simulink model "warplab_mimo_4x4_unconverted_backup"  (Simulink 6.5)
settings: Solver=ode45  StartTime=0.0  StopTime=20000  RelTol=1e-3
libraries: xbsIndex_r4 x197, WARP_Blockset x16
(part 1 of 2)
settings Model: Creator=Melissa.Duarte  LastModifiedBy=melissa.duarte
settings DebuggingCC: MultiTaskDSMMsg=warning  MultiTaskCondExecSysMsg=none
settings RTWCC: IncludeERTFirstTime=on

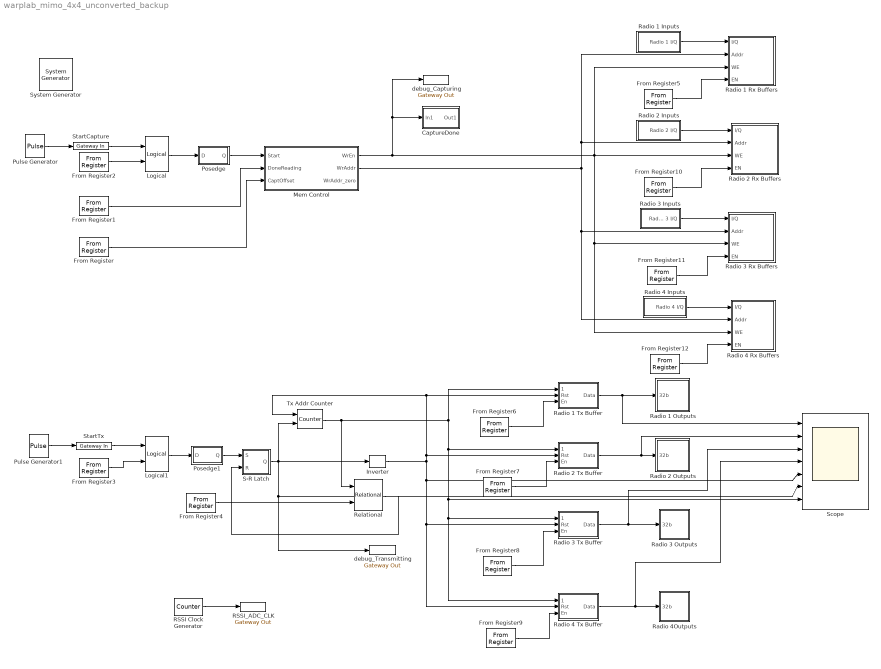
== system warplab_mimo_4x4_unconverted_backup ==
  " System Generator" : xbsIndex_r4/ System Generator  Tag=genX  SystemSampleTime=-1  xilinxfamily=Virtex4  part=xc4vsx35  speed=-10  package=ff668  synthesis_tool=XST  directory=./netlist  testbench=off  simulink_period=1  sysclk_period=10  incr_netlist=off  trim_vbits=Everywhere in SubSystem  dbl_ovrd=According to Block Masks  core_generation=According to Block Masks  run_coregen=off  deprecated_control=off  eval_field=0  block_type=sysgen
      settings: block_version=8.2
  CaptureDone : Subsystem
  From Register : xbsIndex_r4/From Register  shared_memory_name='CaptOffset'  init=100  period=1  ownership=Locally owned and initialized  arith_type=Unsigned  n_bits=14  bin_pt=0  dbl_ovrd=off  block_type=fromreg
      settings: AttributesFormatString=CaptOffset\n<< %<shared_memory_name> >>  infoedit="Register block that reads data to a shared memory register.  Delay of one sample period."  block_version=8.2
  From Register1 : xbsIndex_r4/From Register  shared_memory_name='DoneReading'  init=0  period=1  ownership=Locally owned and initialized  arith_type=Unsigned  n_bits=1  bin_pt=0  dbl_ovrd=off  block_type=fromreg
      settings: AttributesFormatString=DoneReading\n<< %<shared_memory_name> >>  infoedit="Register block that reads data to a shared memory register.  Delay of one sample period."  block_version=8.2
  From Register10 : xbsIndex_r4/From Register  shared_memory_name='RADIO2RXBUFF_RXEN'  init=0  period=1  ownership=Locally owned and initialized  arith_type=Unsigned  n_bits=1  bin_pt=0  dbl_ovrd=off  block_type=fromreg
      settings: AttributesFormatString=RADIO2RXBUFF_RXEN\n<< %<shared_memory_name> >>  infoedit="Register block that reads data to a shared memory register.  Delay of one sample period."  block_version=8.2
  From Register11 : xbsIndex_r4/From Register  shared_memory_name='RADIO3RXBUFF_RXEN'  init=0  period=1  ownership=Locally owned and initialized  arith_type=Unsigned  n_bits=1  bin_pt=0  dbl_ovrd=off  block_type=fromreg
      settings: AttributesFormatString=RADIO3RXBUFF_RXEN\n<< %<shared_memory_name> >>  infoedit="Register block that reads data to a shared memory register.  Delay of one sample period."  block_version=8.2
  From Register12 : xbsIndex_r4/From Register  shared_memory_name='RADIO4RXBUFF_RXEN'  init=0  period=1  ownership=Locally owned and initialized  arith_type=Unsigned  n_bits=1  bin_pt=0  dbl_ovrd=off  block_type=fromreg
      settings: AttributesFormatString=RADIO4RXBUFF_RXEN\n<< %<shared_memory_name> >>  infoedit="Register block that reads data to a shared memory register.  Delay of one sample period."  block_version=8.2
  From Register2 : xbsIndex_r4/From Register  shared_memory_name='StartCapture'  init=0  period=1  ownership=Locally owned and initialized  arith_type=Unsigned  n_bits=1  bin_pt=0  dbl_ovrd=off  block_type=fromreg
      settings: AttributesFormatString=StartCapture\n<< %<shared_memory_name> >>  infoedit="Register block that reads data to a shared memory register.  Delay of one sample period."  block_version=8.2
  From Register3 : xbsIndex_r4/From Register  shared_memory_name='StartTx'  init=0  period=1  ownership=Locally owned and initialized  arith_type=Unsigned  n_bits=1  bin_pt=0  dbl_ovrd=off  block_type=fromreg
      settings: AttributesFormatString=StartTx\n<< %<shared_memory_name> >>  infoedit="Register block that reads data to a shared memory register.  Delay of one sample period."  block_version=8.2
  From Register4 : xbsIndex_r4/From Register  shared_memory_name='TxLength'  init=2^14-1  period=1  ownership=Locally owned and initialized  arith_type=Unsigned  n_bits=14  bin_pt=0  dbl_ovrd=off  block_type=fromreg
      settings: AttributesFormatString=TxLength\n<< %<shared_memory_name> >>  infoedit="Register block that reads data to a shared memory register.  Delay of one sample period."  block_version=8.2
  From Register5 : xbsIndex_r4/From Register  shared_memory_name='RADIO1RXBUFF_RXEN'  init=0  period=1  ownership=Locally owned and initialized  arith_type=Unsigned  n_bits=1  bin_pt=0  dbl_ovrd=off  block_type=fromreg
      settings: AttributesFormatString=RADIO1RXBUFF_RXEN\n<< %<shared_memory_name> >>  infoedit="Register block that reads data to a shared memory register.  Delay of one sample period."  block_version=8.2
  From Register6 : xbsIndex_r4/From Register  shared_memory_name='RADIO1TXBUFF_TXEN'  init=0  period=1  ownership=Locally owned and initialized  arith_type=Unsigned  n_bits=1  bin_pt=0  dbl_ovrd=off  block_type=fromreg
      settings: AttributesFormatString=RADIO1TXBUFF_TXEN\n<< %<shared_memory_name> >>  infoedit="Register block that reads data to a shared memory register.  Delay of one sample period."  block_version=8.2
  From Register7 : xbsIndex_r4/From Register  shared_memory_name='RADIO2TXBUFF_TXEN'  init=0  period=1  ownership=Locally owned and initialized  arith_type=Unsigned  n_bits=1  bin_pt=0  dbl_ovrd=off  block_type=fromreg
      settings: AttributesFormatString=RADIO2TXBUFF_TXEN\n<< %<shared_memory_name> >>  infoedit="Register block that reads data to a shared memory register.  Delay of one sample period."  block_version=8.2
  From Register8 : xbsIndex_r4/From Register  shared_memory_name='RADIO3TXBUFF_TXEN'  init=0  period=1  ownership=Locally owned and initialized  arith_type=Unsigned  n_bits=1  bin_pt=0  dbl_ovrd=off  block_type=fromreg
      settings: AttributesFormatString=RADIO3TXBUFF_TXEN\n<< %<shared_memory_name> >>  infoedit="Register block that reads data to a shared memory register.  Delay of one sample period."  block_version=8.2
  From Register9 : xbsIndex_r4/From Register  shared_memory_name='RADIO4TXBUFF_TXEN'  init=0  period=1  ownership=Locally owned and initialized  arith_type=Unsigned  n_bits=1  bin_pt=0  dbl_ovrd=off  block_type=fromreg
      settings: AttributesFormatString=RADIO4TXBUFF_TXEN\n<< %<shared_memory_name> >>  infoedit="Register block that reads data to a shared memory register.  Delay of one sample period."  block_version=8.2
  Inverter : xbsIndex_r4/Inverter  en=off  latency=0  dbl_ovrd=off  block_type=inv
      settings: block_version=8.2
  Logical : xbsIndex_r4/Logical  logical_function=OR  inputs=2  en=off  latency=0  precision=Full  arith_type=Unsigned  n_bits=16  bin_pt=0  align_bp=on  dbl_ovrd=off  block_type=logical
      settings: block_version=8.2
  Logical1 : xbsIndex_r4/Logical  logical_function=OR  inputs=2  en=off  latency=0  precision=Full  arith_type=Unsigned  n_bits=16  bin_pt=0  align_bp=on  dbl_ovrd=off  block_type=logical
      settings: block_version=8.2
  Mem Control : Subsystem
  Posedge : Subsystem
  Posedge1 : Subsystem
  Pulse Generator : DiscretePulseGenerator  Period=1000000  PulseWidth=50  PhaseDelay=2
  Pulse Generator1 : DiscretePulseGenerator  Period=1000000  PulseWidth=50  PhaseDelay=2
  RSSI Clock Generator : xbsIndex_r4/Counter  cnt_type=Free Running  cnt_to=Inf  operation=Up  start_count=0  cnt_by_val=1  arith_type=Unsigned  n_bits=1  bin_pt=0  load_pin=off  rst=off  en=off  explicit_period=on  period=2  dbl_ovrd=off  use_behavioral_HDL=off  use_rpm=off  block_type=counter
      settings: block_version=VER_STRING_GOES_HERE
  RSSI_ADC_CLK : xbsIndex_r4/Gateway Out  hdl_port=on  timing_constraint=None  locs_specified=off  LOCs={}  block_type=gatewayout
      settings: infoedit="Gateway out block.  Converts Xilinx fixed point inputs into ouputs of type Simulink integer, double, or fixed point.<P><P>Hardware notes:  In hardware these blocks become top level output ports or are discarded, depending on how they are configured."  block_version=8.2
  Radio 1 Rx Buffers : Subsystem
  Radio 1 Tx Buffer : Subsystem
  Radio 1 Inputs : Subsystem
  Radio 1 Outputs : Subsystem
  Radio 2 Rx Buffers : Subsystem
  Radio 2 Tx Buffer : Subsystem
  Radio 2 Inputs : Subsystem
  Radio 2 Outputs : Subsystem
  Radio 3 Rx Buffers : Subsystem
  Radio 3 Tx Buffer : Subsystem
  Radio 3 Inputs : Subsystem
  Radio 3 Outputs : Subsystem
  Radio 4 Rx Buffers : Subsystem
  Radio 4 Tx Buffer : Subsystem
  Radio 4 Inputs : Subsystem
  Radio 4Outputs : Subsystem
  Relational : xbsIndex_r4/Relational  mode=a>=b  en=off  latency=0  dbl_ovrd=off  block_type=relational
      settings: block_version=8.2
  S-R Latch : Subsystem
  Scope : Scope  NumInputPorts=7
      settings: YMin=-5~-5~-5~-5~-5~-5~-5  YMax=5~5~5~5~5~5~5  SaveName=ScopeData2  MaxDataPoints=50000
  StartCapture : xbsIndex_r4/Gateway In  arith_type=Unsigned  n_bits=1  bin_pt=0  quantization="Round  (unbiased: +/- Inf)"  overflow=Saturate  period=1  dbl_ovrd=off  timing_constraint=None  locs_specified=off  LOCs={}  block_type=gatewayin
      settings: infoedit="Gateway in block.  Converts inputs of type Simulink integer, double and fixed point to  Xilinx fixed point type.<P><P>Hardware notes:  In hardware these blocks become top level input ports."  block_version=VER_STRING_GOES_HERE
  StartTx : xbsIndex_r4/Gateway In  arith_type=Unsigned  n_bits=1  bin_pt=0  quantization="Round  (unbiased: +/- Inf)"  overflow=Saturate  period=1  dbl_ovrd=off  timing_constraint=None  locs_specified=off  LOCs={}  block_type=gatewayin
      settings: infoedit="Gateway in block.  Converts inputs of type Simulink integer, double and fixed point to  Xilinx fixed point type.<P><P>Hardware notes:  In hardware these blocks become top level input ports."  block_version=VER_STRING_GOES_HERE
  Tx Addr Counter : xbsIndex_r4/Counter  cnt_type=Free Running  cnt_to=Inf  operation=Up  start_count=0  cnt_by_val=1  arith_type=Unsigned  n_bits=14  bin_pt=0  load_pin=off  rst=on  en=on  explicit_period=off  period=1  dbl_ovrd=off  use_behavioral_HDL=off  use_rpm=off  block_type=counter
      settings: block_version=8.2
  debug_Capturing : xbsIndex_r4/Gateway Out  hdl_port=on  timing_constraint=None  locs_specified=off  LOCs={}  block_type=gatewayout
      settings: infoedit="Gateway out block.  Converts Xilinx fixed point inputs into ouputs of type Simulink integer, double, or fixed point.<P><P>Hardware notes:  In hardware these blocks become top level output ports or are discarded, depending on how they are configured."  block_version=8.2
  debug_Transmitting : xbsIndex_r4/Gateway Out  hdl_port=on  timing_constraint=None  locs_specified=off  LOCs={}  block_type=gatewayout
      settings: infoedit="Gateway out block.  Converts Xilinx fixed point inputs into ouputs of type Simulink integer, double, or fixed point.<P><P>Hardware notes:  In hardware these blocks become top level output ports or are discarded, depending on how they are configured."  block_version=8.2
  wires:
  Posedge/1(Q) -> Mem Control/1(Start)
  From Register/1 -> Mem Control/3(CaptOffset)
  From Register1/1 -> Mem Control/2(DoneReading)
  Pulse Generator/1 -> StartCapture/1
  From Register2/1 -> Logical/2
  Logical/1 -> Posedge/1(D)
  StartCapture/1 -> Logical/1
  Tx Addr Counter/1 -> Relational/1, Radio 1 Tx Buffer/1(RdAddr), Radio 2 Tx Buffer/1(RdAddr), Radio 3 Tx Buffer/1(RdAddr), Radio 4 Tx Buffer/1(RdAddr), Scope/7
  S-R Latch/1(Q) -> Inverter/1, Tx Addr Counter/2, debug_Transmitting/1, Scope/6
  From Register4/1 -> Relational/2
  Relational/1 -> S-R Latch/2(R)
  Inverter/1 -> Radio 1 Tx Buffer/2(Rst), Tx Addr Counter/1, Radio 2 Tx Buffer/2(Rst), Radio 3 Tx Buffer/2(Rst), Radio 4 Tx Buffer/2(Rst), Scope/5
  Radio 1 Inputs/1(Radio 1 I/Q) -> Radio 1 Rx Buffers/1(I/Q)
  RSSI Clock Generator/1 -> RSSI_ADC_CLK/1
  Posedge1/1(Q) -> S-R Latch/1(S)
  Radio 2 Inputs/1(Radio 2 I/Q) -> Radio 2 Rx Buffers/1(I/Q)
  Radio 4 Inputs/1(Radio 4 I/Q) -> Radio 4 Rx Buffers/1(I/Q)
  Radio 3 Inputs/1(Radio 3 I/Q) -> Radio 3 Rx Buffers/1(I/Q)
  Pulse Generator1/1 -> StartTx/1
  StartTx/1 -> Logical1/1
  Logical1/1 -> Posedge1/1(D)
  From Register3/1 -> Logical1/2
  Mem Control/1(WrEn) -> CaptureDone/1(In1), debug_Capturing/1, Radio 2 Rx Buffers/3(WE), Radio 1 Rx Buffers/3(WE), Radio 3 Rx Buffers/3(WE), Radio 4 Rx Buffers/3(WE)
  Mem Control/2(WrAddr) -> Radio 1 Rx Buffers/2(Addr), Radio 2 Rx Buffers/2(Addr), Radio 3 Rx Buffers/2(Addr), Radio 4 Rx Buffers/2(Addr)
  From Register6/1 -> Radio 1 Tx Buffer/3(En)
  From Register7/1 -> Radio 2 Tx Buffer/3(En)
  From Register8/1 -> Radio 3 Tx Buffer/3(En)
  From Register9/1 -> Radio 4 Tx Buffer/3(En)
  From Register5/1 -> Radio 1 Rx Buffers/4(EN)
  From Register10/1 -> Radio 2 Rx Buffers/4(EN)
  From Register11/1 -> Radio 3 Rx Buffers/4(EN)
  From Register12/1 -> Radio 4 Rx Buffers/4(EN)
  Radio 1 Tx Buffer/1(Data) -> Radio 1 Outputs/1(32b), Scope/1
  Radio 2 Tx Buffer/1(Data) -> Radio 2 Outputs/1(32b), Scope/2
  Radio 3 Tx Buffer/1(Data) -> Radio 3 Outputs/1(32b), Scope/3
  Radio 4 Tx Buffer/1(Data) -> Radio 4Outputs/1(32b), Scope/4

== system warplab_mimo_4x4_unconverted_backup/CaptureDone ==
  In1 : Inport
  Inverter1 : xbsIndex_r4/Inverter  en=off  latency=0  dbl_ovrd=off  block_type=inv
      settings: block_version=8.2
  To Register : xbsIndex_r4/To Register  shared_memory_name='CaptureDone'  init=0  ownership=Locally owned and initialized  explicit_data_type=off  arith_type="Signed  (2's comp)"  n_bits=16  bin_pt=14  dbl_ovrd=off  block_type=toreg
      settings: AttributesFormatString=CaptureDone\n<< %<shared_memory_name> >>  infoedit="Register block that writes data to a shared memory register.  Delay of one sample period."  block_version=8.2
  zero3 : xbsIndex_r4/Constant  arith_type=Boolean  const=1  n_bits=1  bin_pt=0  explicit_period=off  period=1  equ=P=C  opselect=C  inp2=PCIN>>17  opr=+  inp1=P  carry=CIN  dbl_ovrd=off  block_type=constant
      settings: block_version=VER_STRING_GOES_HERE
  Out1 : Outport
  wires:
  zero3/1 -> To Register/2
  Inverter1/1 -> To Register/1
  In1/1 -> Inverter1/1
  To Register/1 -> Out1/1

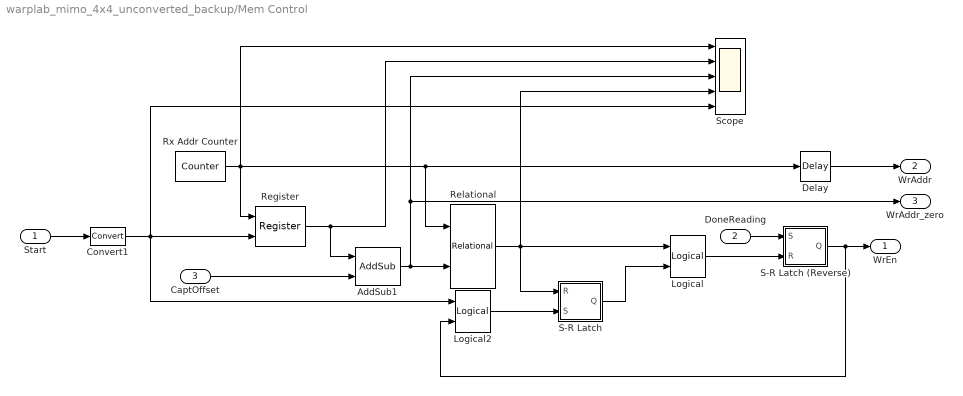
== system warplab_mimo_4x4_unconverted_backup/Mem Control ==
  Start : Inport
  DoneReading : Inport  Port=2
  CaptOffset : Inport  Port=3
  AddSub1 : xbsIndex_r4/AddSub  mode=Subtraction  use_carryin=off  use_carryout=off  en=off  latency=0  precision=User Defined  arith_type=Unsigned  n_bits=14  bin_pt=0  quantization=Truncate  overflow=Wrap  dbl_ovrd=off  use_behavioral_HDL=off  pipelined=off  use_rpm=on  block_type=addsub
      settings: block_version=8.2
  Convert1 : xbsIndex_r4/Convert  arith_type=Boolean  n_bits=16  bin_pt=14  quantization=Truncate  overflow=Wrap  latency=0  dbl_ovrd=off  pipeline=off  block_type=convert
      settings: block_version=8.2
  Delay : xbsIndex_r4/Delay  en=off  latency=1  dbl_ovrd=off  reg_retiming=off  block_type=delay
      settings: infoedit=Hardware notes: A delay line is a chain, each link of which is an SRL16 followed by a flip-flop. If register retiming is enabled, the delay line is a chain of flip-flops.  block_version=8.2
  Logical : xbsIndex_r4/Logical  logical_function=AND  inputs=2  en=off  latency=0  precision=Full  arith_type=Unsigned  n_bits=16  bin_pt=0  align_bp=on  dbl_ovrd=off  block_type=logical
      settings: block_version=8.2
  Logical2 : xbsIndex_r4/Logical  logical_function=AND  inputs=2  en=off  latency=0  precision=Full  arith_type=Unsigned  n_bits=16  bin_pt=0  align_bp=on  dbl_ovrd=off  block_type=logical
      settings: block_version=8.2
  Register : xbsIndex_r4/Register  init=0  rst=off  en=on  dbl_ovrd=off  block_type=register
      settings: block_version=8.2
  Relational : xbsIndex_r4/Relational  mode=a=b  en=off  latency=0  dbl_ovrd=off  block_type=relational
      settings: block_version=8.2
  Rx Addr Counter : xbsIndex_r4/Counter  cnt_type=Free Running  cnt_to=Inf  operation=Up  start_count=0  cnt_by_val=1  arith_type=Unsigned  n_bits=14  bin_pt=0  load_pin=off  rst=off  en=off  explicit_period=on  period=1  dbl_ovrd=off  use_behavioral_HDL=off  use_rpm=off  block_type=counter
      settings: block_version=8.2
  S-R Latch : Subsystem
  S-R Latch (Reverse) : Subsystem
  Scope : Scope  NumInputPorts=5
      settings: TimeRange=100000  YMin=0~-1~15469.8~0~-1  YMax=17500~1~17098.2~1~1
  WrEn : Outport
  WrAddr : Outport  Port=2
  WrAddr_zero : Outport  Port=3
  wires:
  CaptOffset/1 -> AddSub1/2
  Register/1 -> AddSub1/1, Scope/2
  AddSub1/1 -> Relational/2, Scope/3, WrAddr_zero/1
  DoneReading/1 -> S-R Latch (Reverse)/1(S)
  Relational/1 -> S-R Latch/1(R), Logical/1, Scope/4
  Rx Addr Counter/1 -> Scope/1, Register/1, Delay/1, Relational/1
  Start/1 -> Convert1/1
  S-R Latch (Reverse)/1(Q) -> WrEn/1, Logical2/2
  Delay/1 -> WrAddr/1
  Convert1/1 -> Register/2, Scope/5, Logical2/1
  Logical/1 -> S-R Latch (Reverse)/2(R)
  S-R Latch/1(Q) -> Logical/2
  Logical2/1 -> S-R Latch/2(S)

== system warplab_mimo_4x4_unconverted_backup/Posedge ==
  D : Inport
  Delay : xbsIndex_r4/Delay  en=off  latency=1  dbl_ovrd=off  reg_retiming=off  block_type=delay
      settings: infoedit=Hardware notes: A delay line is a chain, each link of which is an SRL16 followed by a flip-flop. If register retiming is enabled, the delay line is a chain of flip-flops.  block_version=8.2
  Inverter : xbsIndex_r4/Inverter  en=off  latency=0  dbl_ovrd=off  block_type=inv
      settings: block_version=8.2
  Logical : xbsIndex_r4/Logical  logical_function=AND  inputs=2  en=off  latency=0  precision=Full  arith_type=Unsigned  n_bits=16  bin_pt=0  align_bp=on  dbl_ovrd=off  block_type=logical
      settings: block_version=8.2
  Q : Outport
  wires:
  D/1 -> Inverter/1, Logical/1
  Inverter/1 -> Delay/1
  Delay/1 -> Logical/2
  Logical/1 -> Q/1

== system warplab_mimo_4x4_unconverted_backup/Posedge1 ==
  D : Inport
  Delay : xbsIndex_r4/Delay  en=off  latency=1  dbl_ovrd=off  reg_retiming=off  block_type=delay
      settings: infoedit=Hardware notes: A delay line is a chain, each link of which is an SRL16 followed by a flip-flop. If register retiming is enabled, the delay line is a chain of flip-flops.  block_version=8.2
  Inverter : xbsIndex_r4/Inverter  en=off  latency=0  dbl_ovrd=off  block_type=inv
      settings: block_version=8.2
  Logical : xbsIndex_r4/Logical  logical_function=AND  inputs=2  en=off  latency=0  precision=Full  arith_type=Unsigned  n_bits=16  bin_pt=0  align_bp=on  dbl_ovrd=off  block_type=logical
      settings: block_version=8.2
  Q : Outport
  wires:
  Logical/1 -> Q/1
  Delay/1 -> Logical/2
  Inverter/1 -> Delay/1
  D/1 -> Logical/1, Inverter/1

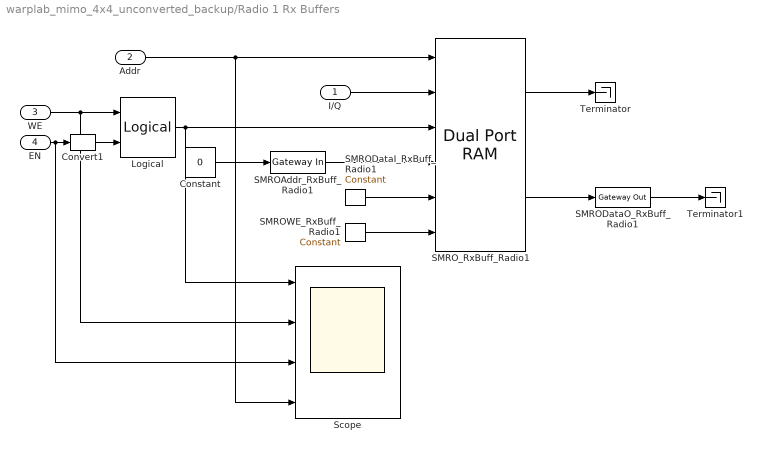
== system warplab_mimo_4x4_unconverted_backup/Radio 1 Rx Buffers ==
  I/Q : Inport
  Addr : Inport  Port=2
  WE : Inport  Port=3
  EN : Inport  Port=4
  Constant : Constant  Value=0  OutDataType=sfix(16)  ConRadixGroup=Use specified scaling  OutScaling=2^0  SampleTime=inf  FramePeriod=inf
  Convert1 : xbsIndex_r4/Convert  arith_type=Boolean  n_bits=16  bin_pt=14  quantization=Truncate  overflow=Wrap  latency=0  dbl_ovrd=off  pipeline=off  block_type=convert
      settings: block_version=8.2
  Logical : xbsIndex_r4/Logical  logical_function=AND  inputs=2  en=off  latency=0  precision=Full  arith_type=Unsigned  n_bits=16  bin_pt=0  align_bp=on  dbl_ovrd=off  block_type=logical
      settings: block_version=9.1.01
  SMROAddr_RxBuff_Radio1 : xbsIndex_r4/Gateway In  arith_type=Unsigned  n_bits=14  bin_pt=0  quantization="Round  (unbiased: +/- Inf)"  overflow=Saturate  period=1  dbl_ovrd=off  timing_constraint=None  locs_specified=off  LOCs={}  block_type=gatewayin
      settings: infoedit="Gateway in block.  Converts inputs of type Simulink integer, double and fixed point to  Xilinx fixed point type.<P><P>Hardware notes:  In hardware these blocks become top level input ports."  block_version=VER_STRING_GOES_HERE
  SMRODataI_RxBuff_Radio1 : xbsIndex_r4/Constant  arith_type=Unsigned  const=0  n_bits=32  bin_pt=0  explicit_period=off  period=1  equ=P=C  opselect=C  inp2=PCIN>>17  opr=+  inp1=P  carry=CIN  dbl_ovrd=off  block_type=constant
      settings: block_version=VER_STRING_GOES_HERE
  SMRODataO_RxBuff_Radio1 : xbsIndex_r4/Gateway Out  hdl_port=on  timing_constraint=None  locs_specified=off  LOCs={}  block_type=gatewayout
      settings: infoedit="Gateway out block.  Converts Xilinx fixed point inputs into ouputs of type Simulink integer, double, or fixed point.<P><P>Hardware notes:  In hardware these blocks become top level output ports or are discarded, depending on how they are configured."  xl_area=[0, 0, 0, 0, 0, 0, 0]  block_version=VER_STRING_GOES_HERE
  SMROWE_RxBuff_Radio1 : xbsIndex_r4/Constant  arith_type=Boolean  const=0  n_bits=3  bin_pt=0  explicit_period=off  period=1  equ=P=C  opselect=C  inp2=PCIN>>17  opr=+  inp1=P  carry=CIN  dbl_ovrd=off  block_type=constant
      settings: block_version=VER_STRING_GOES_HERE
  SMRO_RxBuff_Radio1 : xbsIndex_r4/Dual Port RAM  depth=2^14  initVector=1:2^14  distributed_mem=Block RAM  init_a=0  init_b=0  rst_a=off  rst_b=off  en_a=off  en_b=off  latency=1  write_mode_A=Read After Write  write_mode_B=Read After Write  dbl_ovrd=off  optimize=Area  use_rpm=on  block_type=dpram
      settings: block_version=VER_STRING_GOES_HERE
  Scope : Scope  NumInputPorts=4
      settings: YMin=-5~-5~-5~-5  YMax=5~5~5~5  SaveName=ScopeData3  MaxDataPoints=50000
  Terminator : Terminator
  Terminator1 : Terminator
  wires:
  I/Q/1 -> SMRO_RxBuff_Radio1/2
  Addr/1 -> SMRO_RxBuff_Radio1/1, Scope/4
  SMRODataO_RxBuff_Radio1/1 -> Terminator1/1
  SMRO_RxBuff_Radio1/1 -> Terminator/1
  SMROAddr_RxBuff_Radio1/1 -> SMRO_RxBuff_Radio1/4
  SMRO_RxBuff_Radio1/2 -> SMRODataO_RxBuff_Radio1/1
  Constant/1 -> SMROAddr_RxBuff_Radio1/1
  SMRODataI_RxBuff_Radio1/1 -> SMRO_RxBuff_Radio1/5
  SMROWE_RxBuff_Radio1/1 -> SMRO_RxBuff_Radio1/6
  Logical/1 -> SMRO_RxBuff_Radio1/3, Scope/1
  WE/1 -> Logical/1, Scope/2
  EN/1 -> Convert1/1, Scope/3
  Convert1/1 -> Logical/2

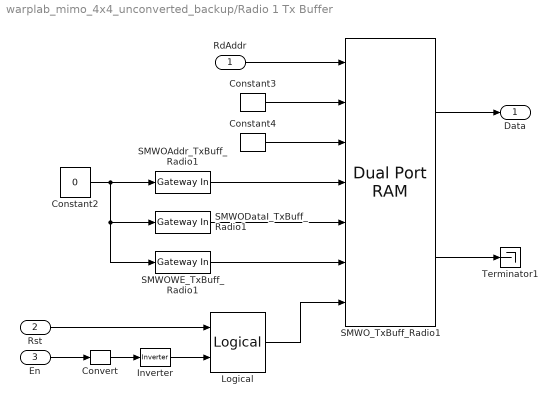
== system warplab_mimo_4x4_unconverted_backup/Radio 1 Tx Buffer ==
  RdAddr : Inport
  Rst : Inport  Port=2
  En : Inport  Port=3
  Constant2 : Constant  Value=0  OutDataType=sfix(16)  ConRadixGroup=Use specified scaling  OutScaling=2^0  SampleTime=inf  FramePeriod=inf
  Constant3 : xbsIndex_r4/Constant  arith_type=Unsigned  const=0  n_bits=32  bin_pt=0  explicit_period=off  period=1  equ=P=C  opselect=C  inp2=PCIN>>17  opr=+  inp1=P  carry=CIN  dbl_ovrd=off  block_type=constant
      settings: block_version=VER_STRING_GOES_HERE
  Constant4 : xbsIndex_r4/Constant  arith_type=Boolean  const=0  n_bits=1  bin_pt=0  explicit_period=off  period=1  equ=P=C  opselect=C  inp2=PCIN>>17  opr=+  inp1=P  carry=CIN  dbl_ovrd=off  block_type=constant
      settings: block_version=VER_STRING_GOES_HERE
  Convert : xbsIndex_r4/Convert  arith_type=Boolean  n_bits=16  bin_pt=14  quantization=Truncate  overflow=Wrap  latency=0  dbl_ovrd=off  pipeline=off  block_type=convert
      settings: block_version=8.2
  Inverter : xbsIndex_r4/Inverter  en=off  latency=0  dbl_ovrd=off  block_type=inv
      settings: block_version=9.1.01
  Logical : xbsIndex_r4/Logical  logical_function=OR  inputs=2  en=off  latency=0  precision=Full  arith_type=Unsigned  n_bits=16  bin_pt=0  align_bp=on  dbl_ovrd=off  block_type=logical
      settings: block_version=9.1.01
  SMWOAddr_TxBuff_Radio1 : xbsIndex_r4/Gateway In  arith_type=Unsigned  n_bits=14  bin_pt=0  quantization="Round  (unbiased: +/- Inf)"  overflow=Saturate  period=1  dbl_ovrd=off  timing_constraint=None  locs_specified=off  LOCs={}  block_type=gatewayin
      settings: infoedit="Gateway in block.  Converts inputs of type Simulink integer, double and fixed point to  Xilinx fixed point type.<P><P>Hardware notes:  In hardware these blocks become top level input ports."  block_version=VER_STRING_GOES_HERE
  SMWODataI_TxBuff_Radio1 : xbsIndex_r4/Gateway In  arith_type=Unsigned  n_bits=32  bin_pt=0  quantization="Round  (unbiased: +/- Inf)"  overflow=Saturate  period=1  dbl_ovrd=off  timing_constraint=None  locs_specified=off  LOCs={}  block_type=gatewayin
      settings: infoedit="Gateway in block.  Converts inputs of type Simulink integer, double and fixed point to  Xilinx fixed point type.<P><P>Hardware notes:  In hardware these blocks become top level input ports."  block_version=VER_STRING_GOES_HERE
  SMWOWE_TxBuff_Radio1 : xbsIndex_r4/Gateway In  arith_type=Boolean  n_bits=1  bin_pt=0  quantization="Round  (unbiased: +/- Inf)"  overflow=Saturate  period=1  dbl_ovrd=off  timing_constraint=None  locs_specified=off  LOCs={}  block_type=gatewayin
      settings: infoedit="Gateway in block.  Converts inputs of type Simulink integer, double and fixed point to  Xilinx fixed point type.<P><P>Hardware notes:  In hardware these blocks become top level input ports."  block_version=VER_STRING_GOES_HERE
  SMWO_TxBuff_Radio1 : xbsIndex_r4/Dual Port RAM  depth=2^14  initVector=1:2^14  distributed_mem=Block RAM  init_a=0  init_b=0  rst_a=on  rst_b=off  en_a=off  en_b=off  latency=1  write_mode_A=Read After Write  write_mode_B=Read After Write  dbl_ovrd=off  optimize=Area  use_rpm=on  block_type=dpram
      settings: block_version=VER_STRING_GOES_HERE
  Terminator1 : Terminator
  Data : Outport
  wires:
  SMWO_TxBuff_Radio1/2 -> Terminator1/1
  SMWODataI_TxBuff_Radio1/1 -> SMWO_TxBuff_Radio1/5
  SMWOWE_TxBuff_Radio1/1 -> SMWO_TxBuff_Radio1/6
  SMWOAddr_TxBuff_Radio1/1 -> SMWO_TxBuff_Radio1/4
  Constant3/1 -> SMWO_TxBuff_Radio1/2
  Constant4/1 -> SMWO_TxBuff_Radio1/3
  Constant2/1 -> SMWOAddr_TxBuff_Radio1/1, SMWODataI_TxBuff_Radio1/1, SMWOWE_TxBuff_Radio1/1
  RdAddr/1 -> SMWO_TxBuff_Radio1/1
  SMWO_TxBuff_Radio1/1 -> Data/1
  Logical/1 -> SMWO_TxBuff_Radio1/7
  Rst/1 -> Logical/1
  Inverter/1 -> Logical/2
  En/1 -> Convert/1
  Convert/1 -> Inverter/1

== system warplab_mimo_4x4_unconverted_backup/Radio 1 Inputs ==
  ADC I : Subsystem
  ADC Q : Subsystem
  Concatenates_1 : Subsystem
  Scope : Scope  NumInputPorts=3
      settings: YMin=-5~-5~-5  YMax=5~5~5
  Radio 1 I/Q : Outport
  wires:
  ADC Q/2(ADC Q) -> Concatenates_1/4(ADC_Q), Scope/2
  ADC Q/1(OTR Q) -> Concatenates_1/3(OTR_Q)
  ADC I/2(ADC I) -> Concatenates_1/2(ADC_I), Scope/1
  ADC I/1(OTR I) -> Concatenates_1/1(OTR_I)
  Concatenates_1/1(32b) -> Radio 1 I/Q/1

== system warplab_mimo_4x4_unconverted_backup/Radio 1 Outputs ==
  32b : Inport
  16LSB : xbsIndex_r4/Slice  nbits=16  boolean_output=off  mode=Lower Bit Location + Width  bit1=0  base1=MSB of Input  bit0=0  base0=LSB of Input  dbl_ovrd=off  block_type=slice
      settings: infoedit="Extracts a given range of bits from each input sample and presents it at the output.  The output type is ordinarily unsigned with binary point at zero, but can be Boolean when the slice is one bit wide.<P><P>Hardware notes: In hardware this block costs nothing."  block_version=8.2
  16MSB : xbsIndex_r4/Slice  nbits=16  boolean_output=off  mode=Upper Bit Location + Width  bit1=0  base1=MSB of Input  bit0=0  base0=LSB of Input  dbl_ovrd=off  block_type=slice
      settings: infoedit="Extracts a given range of bits from each input sample and presents it at the output.  The output type is ordinarily unsigned with binary point at zero, but can be Boolean when the slice is one bit wide.<P><P>Hardware notes: In hardware this block costs nothing."  block_version=8.2
  Radio 1 DAC I : WARP_Blockset/WARP Radio ADC//DACs/Radio 1 DAC I  SystemSampleTime=-1
  Radio 1 DAC Q : WARP_Blockset/WARP Radio ADC//DACs/Radio 1 DAC Q  SystemSampleTime=-1
  Register : xbsIndex_r4/Register  init=0  rst=off  en=off  dbl_ovrd=off  block_type=register
      settings: block_version=8.2
  Register1 : xbsIndex_r4/Register  init=0  rst=off  en=off  dbl_ovrd=off  block_type=register
      settings: block_version=8.2
  Reinterpret : xbsIndex_r4/Reinterpret  force_arith_type=on  arith_type="Signed  (2's comp)"  force_bin_pt=on  bin_pt=15  block_type=reinterpret
      settings: infoedit="Changes signal type without altering the binary representation.   You can changed the signal between signed and unsigned, and relocate the binary point.<P><P>Hardware notes: In hardware this block costs nothing.<P><P>Example:  Suppose the input is 6 bits wide, signed, with 2 fractional bits, and the output is forced to unsigned with 0 fractional bits.  Then an input of -2.0 (1110.00 in binary 2's complement) becomes an output of 56 (111000 in binary)."  block_version=8.2
  Reinterpret1 : xbsIndex_r4/Reinterpret  force_arith_type=on  arith_type="Signed  (2's comp)"  force_bin_pt=on  bin_pt=15  block_type=reinterpret
      settings: infoedit="Changes signal type without altering the binary representation.   You can changed the signal between signed and unsigned, and relocate the binary point.<P><P>Hardware notes: In hardware this block costs nothing.<P><P>Example:  Suppose the input is 6 bits wide, signed, with 2 fractional bits, and the output is forced to unsigned with 0 fractional bits.  Then an input of -2.0 (1110.00 in binary 2's complement) becomes an output of 56 (111000 in binary)."  block_version=8.2
  Terminator1 : Terminator
  Terminator2 : Terminator
  wires:
  Register1/1 -> Radio 1 DAC Q/1
  Register/1 -> Radio 1 DAC I/1
  16MSB/1 -> Reinterpret/1
  16LSB/1 -> Reinterpret1/1
  Reinterpret/1 -> Register/1
  Reinterpret1/1 -> Register1/1
  Radio 1 DAC I/1 -> Terminator1/1
  Radio 1 DAC Q/1 -> Terminator2/1
  32b/1 -> 16LSB/1, 16MSB/1

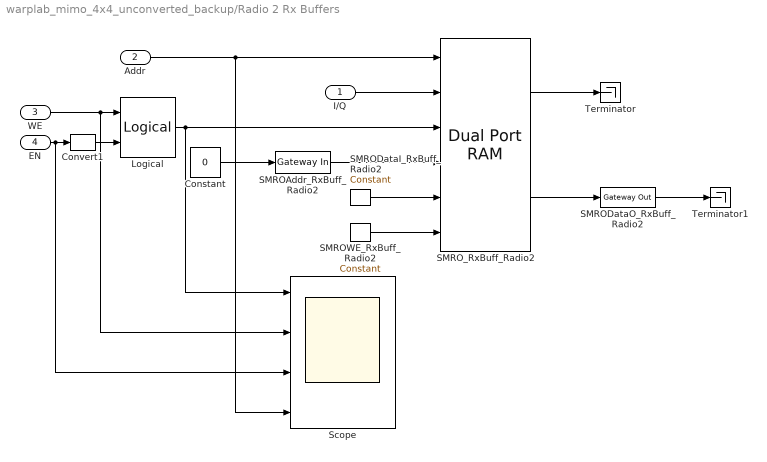
== system warplab_mimo_4x4_unconverted_backup/Radio 2 Rx Buffers ==
  I/Q : Inport
  Addr : Inport  Port=2
  WE : Inport  Port=3
  EN : Inport  Port=4
  Constant : Constant  Value=0  OutDataType=sfix(16)  ConRadixGroup=Use specified scaling  OutScaling=2^0  SampleTime=inf  FramePeriod=inf
  Convert1 : xbsIndex_r4/Convert  arith_type=Boolean  n_bits=16  bin_pt=14  quantization=Truncate  overflow=Wrap  latency=0  dbl_ovrd=off  pipeline=off  block_type=convert
      settings: block_version=8.2
  Logical : xbsIndex_r4/Logical  logical_function=AND  inputs=2  en=off  latency=0  precision=Full  arith_type=Unsigned  n_bits=16  bin_pt=0  align_bp=on  dbl_ovrd=off  block_type=logical
      settings: block_version=9.1.01
  SMROAddr_RxBuff_Radio2 : xbsIndex_r4/Gateway In  arith_type=Unsigned  n_bits=14  bin_pt=0  quantization="Round  (unbiased: +/- Inf)"  overflow=Saturate  period=1  dbl_ovrd=off  timing_constraint=None  locs_specified=off  LOCs={}  block_type=gatewayin
      settings: infoedit="Gateway in block.  Converts inputs of type Simulink integer, double and fixed point to  Xilinx fixed point type.<P><P>Hardware notes:  In hardware these blocks become top level input ports."  block_version=VER_STRING_GOES_HERE
  SMRODataI_RxBuff_Radio2 : xbsIndex_r4/Constant  arith_type=Unsigned  const=0  n_bits=32  bin_pt=0  explicit_period=off  period=1  equ=P=C  opselect=C  inp2=PCIN>>17  opr=+  inp1=P  carry=CIN  dbl_ovrd=off  block_type=constant
      settings: block_version=VER_STRING_GOES_HERE
  SMRODataO_RxBuff_Radio2 : xbsIndex_r4/Gateway Out  hdl_port=on  timing_constraint=None  locs_specified=off  LOCs={}  block_type=gatewayout
      settings: infoedit="Gateway out block.  Converts Xilinx fixed point inputs into ouputs of type Simulink integer, double, or fixed point.<P><P>Hardware notes:  In hardware these blocks become top level output ports or are discarded, depending on how they are configured."  xl_area=[0, 0, 0, 0, 0, 0, 0]  block_version=VER_STRING_GOES_HERE
  SMROWE_RxBuff_Radio2 : xbsIndex_r4/Constant  arith_type=Boolean  const=0  n_bits=3  bin_pt=0  explicit_period=off  period=1  equ=P=C  opselect=C  inp2=PCIN>>17  opr=+  inp1=P  carry=CIN  dbl_ovrd=off  block_type=constant
      settings: block_version=VER_STRING_GOES_HERE
  SMRO_RxBuff_Radio2 : xbsIndex_r4/Dual Port RAM  depth=2^14  initVector=1:2^14  distributed_mem=Block RAM  init_a=0  init_b=0  rst_a=off  rst_b=off  en_a=off  en_b=off  latency=1  write_mode_A=Read After Write  write_mode_B=Read After Write  dbl_ovrd=off  optimize=Area  use_rpm=on  block_type=dpram
      settings: block_version=VER_STRING_GOES_HERE
  Scope : Scope  NumInputPorts=4
      settings: YMin=-5~-5~-5~-5  YMax=5~5~5~5  SaveName=ScopeData4  MaxDataPoints=50000
  Terminator : Terminator
  Terminator1 : Terminator
  wires:
  I/Q/1 -> SMRO_RxBuff_Radio2/2
  Addr/1 -> SMRO_RxBuff_Radio2/1, Scope/4
  SMRODataO_RxBuff_Radio2/1 -> Terminator1/1
  SMRO_RxBuff_Radio2/1 -> Terminator/1
  SMROAddr_RxBuff_Radio2/1 -> SMRO_RxBuff_Radio2/4
  SMRO_RxBuff_Radio2/2 -> SMRODataO_RxBuff_Radio2/1
  Constant/1 -> SMROAddr_RxBuff_Radio2/1
  SMRODataI_RxBuff_Radio2/1 -> SMRO_RxBuff_Radio2/5
  SMROWE_RxBuff_Radio2/1 -> SMRO_RxBuff_Radio2/6
  Logical/1 -> SMRO_RxBuff_Radio2/3, Scope/1
  WE/1 -> Logical/1, Scope/2
  EN/1 -> Convert1/1, Scope/3
  Convert1/1 -> Logical/2

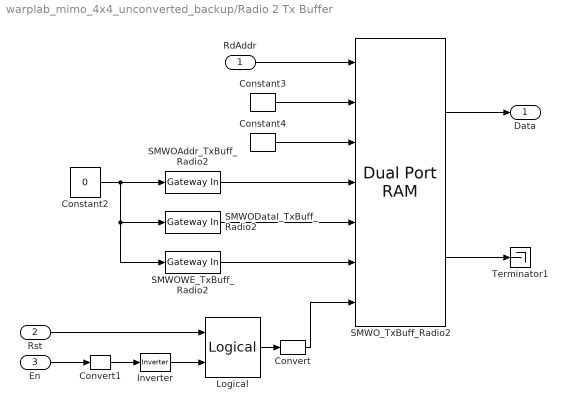
== system warplab_mimo_4x4_unconverted_backup/Radio 2 Tx Buffer ==
  RdAddr : Inport
  Rst : Inport  Port=2
  En : Inport  Port=3
  Constant2 : Constant  Value=0  OutDataType=sfix(16)  ConRadixGroup=Use specified scaling  OutScaling=2^0  SampleTime=inf  FramePeriod=inf
  Constant3 : xbsIndex_r4/Constant  arith_type=Unsigned  const=0  n_bits=32  bin_pt=0  explicit_period=off  period=1  equ=P=C  opselect=C  inp2=PCIN>>17  opr=+  inp1=P  carry=CIN  dbl_ovrd=off  block_type=constant
      settings: block_version=VER_STRING_GOES_HERE
  Constant4 : xbsIndex_r4/Constant  arith_type=Boolean  const=0  n_bits=1  bin_pt=0  explicit_period=off  period=1  equ=P=C  opselect=C  inp2=PCIN>>17  opr=+  inp1=P  carry=CIN  dbl_ovrd=off  block_type=constant
      settings: block_version=VER_STRING_GOES_HERE
  Convert : xbsIndex_r4/Convert  arith_type=Boolean  n_bits=16  bin_pt=14  quantization=Truncate  overflow=Wrap  latency=0  dbl_ovrd=off  pipeline=off  block_type=convert
      settings: block_version=8.2
  Convert1 : xbsIndex_r4/Convert  arith_type=Boolean  n_bits=16  bin_pt=14  quantization=Truncate  overflow=Wrap  latency=0  dbl_ovrd=off  pipeline=off  block_type=convert
      settings: block_version=8.2
  Inverter : xbsIndex_r4/Inverter  en=off  latency=0  dbl_ovrd=off  block_type=inv
      settings: block_version=9.1.01
  Logical : xbsIndex_r4/Logical  logical_function=OR  inputs=2  en=off  latency=0  precision=Full  arith_type=Unsigned  n_bits=16  bin_pt=0  align_bp=on  dbl_ovrd=off  block_type=logical
      settings: block_version=9.1.01
  SMWOAddr_TxBuff_Radio2 : xbsIndex_r4/Gateway In  arith_type=Unsigned  n_bits=14  bin_pt=0  quantization="Round  (unbiased: +/- Inf)"  overflow=Saturate  period=1  dbl_ovrd=off  timing_constraint=None  locs_specified=off  LOCs={}  block_type=gatewayin
      settings: infoedit="Gateway in block.  Converts inputs of type Simulink integer, double and fixed point to  Xilinx fixed point type.<P><P>Hardware notes:  In hardware these blocks become top level input ports."  block_version=VER_STRING_GOES_HERE
  SMWODataI_TxBuff_Radio2 : xbsIndex_r4/Gateway In  arith_type=Unsigned  n_bits=32  bin_pt=0  quantization="Round  (unbiased: +/- Inf)"  overflow=Saturate  period=1  dbl_ovrd=off  timing_constraint=None  locs_specified=off  LOCs={}  block_type=gatewayin
      settings: infoedit="Gateway in block.  Converts inputs of type Simulink integer, double and fixed point to  Xilinx fixed point type.<P><P>Hardware notes:  In hardware these blocks become top level input ports."  block_version=VER_STRING_GOES_HERE
  SMWOWE_TxBuff_Radio2 : xbsIndex_r4/Gateway In  arith_type=Boolean  n_bits=1  bin_pt=0  quantization="Round  (unbiased: +/- Inf)"  overflow=Saturate  period=1  dbl_ovrd=off  timing_constraint=None  locs_specified=off  LOCs={}  block_type=gatewayin
      settings: infoedit="Gateway in block.  Converts inputs of type Simulink integer, double and fixed point to  Xilinx fixed point type.<P><P>Hardware notes:  In hardware these blocks become top level input ports."  block_version=VER_STRING_GOES_HERE
  SMWO_TxBuff_Radio2 : xbsIndex_r4/Dual Port RAM  depth=2^14  initVector=1:2^14  distributed_mem=Block RAM  init_a=0  init_b=0  rst_a=on  rst_b=off  en_a=off  en_b=off  latency=1  write_mode_A=Read After Write  write_mode_B=Read After Write  dbl_ovrd=off  optimize=Area  use_rpm=on  block_type=dpram
      settings: block_version=VER_STRING_GOES_HERE
  Terminator1 : Terminator
  Data : Outport
  wires:
  SMWO_TxBuff_Radio2/2 -> Terminator1/1
  SMWODataI_TxBuff_Radio2/1 -> SMWO_TxBuff_Radio2/5
  SMWOWE_TxBuff_Radio2/1 -> SMWO_TxBuff_Radio2/6
  SMWOAddr_TxBuff_Radio2/1 -> SMWO_TxBuff_Radio2/4
  Constant3/1 -> SMWO_TxBuff_Radio2/2
  Constant4/1 -> SMWO_TxBuff_Radio2/3
  Constant2/1 -> SMWOAddr_TxBuff_Radio2/1, SMWODataI_TxBuff_Radio2/1, SMWOWE_TxBuff_Radio2/1
  RdAddr/1 -> SMWO_TxBuff_Radio2/1
  SMWO_TxBuff_Radio2/1 -> Data/1
  Logical/1 -> Convert/1
  Convert/1 -> SMWO_TxBuff_Radio2/7
  Rst/1 -> Logical/1
  En/1 -> Convert1/1
  Convert1/1 -> Inverter/1
  Inverter/1 -> Logical/2

== system warplab_mimo_4x4_unconverted_backup/Radio 2 Inputs ==
  ADC I : Subsystem
  ADC Q : Subsystem
  Concatenates_1 : Subsystem
  Scope : Scope  NumInputPorts=3
      settings: YMin=-5~-5~-5  YMax=5~5~5
  Radio 2 I/Q : Outport
  wires:
  ADC Q/2(ADC Q) -> Concatenates_1/4(ADC_Q), Scope/2
  ADC Q/1(OTR Q) -> Concatenates_1/3(OTR_Q)
  ADC I/2(ADC I) -> Concatenates_1/2(ADC_I), Scope/1
  ADC I/1(OTR I) -> Concatenates_1/1(OTR_I)
  Concatenates_1/1(32b) -> Radio 2 I/Q/1

== system warplab_mimo_4x4_unconverted_backup/Radio 2 Outputs ==
  32b : Inport
  16LSB : xbsIndex_r4/Slice  nbits=16  boolean_output=off  mode=Lower Bit Location + Width  bit1=0  base1=MSB of Input  bit0=0  base0=LSB of Input  dbl_ovrd=off  block_type=slice
      settings: infoedit="Extracts a given range of bits from each input sample and presents it at the output.  The output type is ordinarily unsigned with binary point at zero, but can be Boolean when the slice is one bit wide.<P><P>Hardware notes: In hardware this block costs nothing."  block_version=8.2
  16MSB : xbsIndex_r4/Slice  nbits=16  boolean_output=off  mode=Upper Bit Location + Width  bit1=0  base1=MSB of Input  bit0=0  base0=LSB of Input  dbl_ovrd=off  block_type=slice
      settings: infoedit="Extracts a given range of bits from each input sample and presents it at the output.  The output type is ordinarily unsigned with binary point at zero, but can be Boolean when the slice is one bit wide.<P><P>Hardware notes: In hardware this block costs nothing."  block_version=8.2
  Radio 2 DAC I : WARP_Blockset/WARP Radio ADC//DACs/Radio 2 DAC I  SystemSampleTime=-1
  Radio 2 DAC Q : WARP_Blockset/WARP Radio ADC//DACs/Radio 2 DAC Q  SystemSampleTime=-1
  Register : xbsIndex_r4/Register  init=0  rst=off  en=off  dbl_ovrd=off  block_type=register
      settings: block_version=8.2
  Register1 : xbsIndex_r4/Register  init=0  rst=off  en=off  dbl_ovrd=off  block_type=register
      settings: block_version=8.2
  Reinterpret : xbsIndex_r4/Reinterpret  force_arith_type=on  arith_type="Signed  (2's comp)"  force_bin_pt=on  bin_pt=15  block_type=reinterpret
      settings: infoedit="Changes signal type without altering the binary representation.   You can changed the signal between signed and unsigned, and relocate the binary point.<P><P>Hardware notes: In hardware this block costs nothing.<P><P>Example:  Suppose the input is 6 bits wide, signed, with 2 fractional bits, and the output is forced to unsigned with 0 fractional bits.  Then an input of -2.0 (1110.00 in binary 2's complement) becomes an output of 56 (111000 in binary)."  block_version=8.2
  Reinterpret1 : xbsIndex_r4/Reinterpret  force_arith_type=on  arith_type="Signed  (2's comp)"  force_bin_pt=on  bin_pt=15  block_type=reinterpret
      settings: infoedit="Changes signal type without altering the binary representation.   You can changed the signal between signed and unsigned, and relocate the binary point.<P><P>Hardware notes: In hardware this block costs nothing.<P><P>Example:  Suppose the input is 6 bits wide, signed, with 2 fractional bits, and the output is forced to unsigned with 0 fractional bits.  Then an input of -2.0 (1110.00 in binary 2's complement) becomes an output of 56 (111000 in binary)."  block_version=8.2
  Terminator1 : Terminator
  Terminator2 : Terminator
  wires:
  Radio 2 DAC Q/1 -> Terminator2/1
  Radio 2 DAC I/1 -> Terminator1/1
  Reinterpret1/1 -> Register1/1
  Reinterpret/1 -> Register/1
  16LSB/1 -> Reinterpret1/1
  16MSB/1 -> Reinterpret/1
  Register/1 -> Radio 2 DAC I/1
  Register1/1 -> Radio 2 DAC Q/1
  32b/1 -> 16MSB/1, 16LSB/1

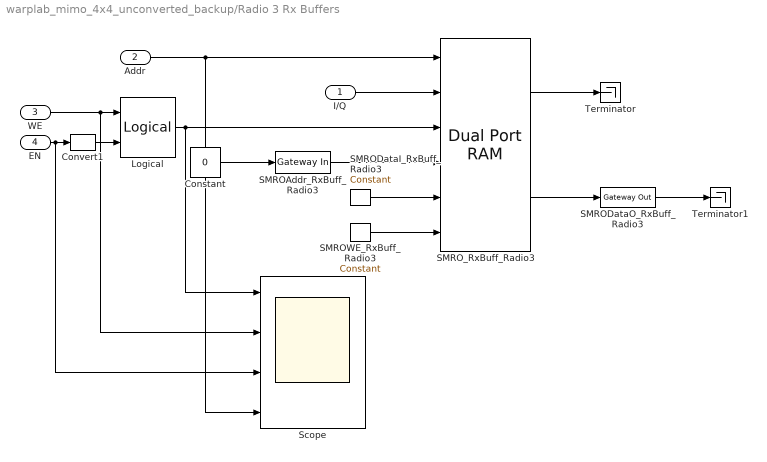
== system warplab_mimo_4x4_unconverted_backup/Radio 3 Rx Buffers ==
  I/Q : Inport
  Addr : Inport  Port=2
  WE : Inport  Port=3
  EN : Inport  Port=4
  Constant : Constant  Value=0  OutDataType=sfix(16)  ConRadixGroup=Use specified scaling  OutScaling=2^0  SampleTime=inf  FramePeriod=inf
  Convert1 : xbsIndex_r4/Convert  arith_type=Boolean  n_bits=16  bin_pt=14  quantization=Truncate  overflow=Wrap  latency=0  dbl_ovrd=off  pipeline=off  block_type=convert
      settings: block_version=8.2
  Logical : xbsIndex_r4/Logical  logical_function=AND  inputs=2  en=off  latency=0  precision=Full  arith_type=Unsigned  n_bits=16  bin_pt=0  align_bp=on  dbl_ovrd=off  block_type=logical
      settings: block_version=9.1.01
  SMROAddr_RxBuff_Radio3 : xbsIndex_r4/Gateway In  arith_type=Unsigned  n_bits=14  bin_pt=0  quantization="Round  (unbiased: +/- Inf)"  overflow=Saturate  period=1  dbl_ovrd=off  timing_constraint=None  locs_specified=off  LOCs={}  block_type=gatewayin
      settings: infoedit="Gateway in block.  Converts inputs of type Simulink integer, double and fixed point to  Xilinx fixed point type.<P><P>Hardware notes:  In hardware these blocks become top level input ports."  block_version=VER_STRING_GOES_HERE
  SMRODataI_RxBuff_Radio3 : xbsIndex_r4/Constant  arith_type=Unsigned  const=0  n_bits=32  bin_pt=0  explicit_period=off  period=1  equ=P=C  opselect=C  inp2=PCIN>>17  opr=+  inp1=P  carry=CIN  dbl_ovrd=off  block_type=constant
      settings: block_version=VER_STRING_GOES_HERE
  SMRODataO_RxBuff_Radio3 : xbsIndex_r4/Gateway Out  hdl_port=on  timing_constraint=None  locs_specified=off  LOCs={}  block_type=gatewayout
      settings: infoedit="Gateway out block.  Converts Xilinx fixed point inputs into ouputs of type Simulink integer, double, or fixed point.<P><P>Hardware notes:  In hardware these blocks become top level output ports or are discarded, depending on how they are configured."  xl_area=[0, 0, 0, 0, 0, 0, 0]  block_version=VER_STRING_GOES_HERE
  SMROWE_RxBuff_Radio3 : xbsIndex_r4/Constant  arith_type=Boolean  const=0  n_bits=3  bin_pt=0  explicit_period=off  period=1  equ=P=C  opselect=C  inp2=PCIN>>17  opr=+  inp1=P  carry=CIN  dbl_ovrd=off  block_type=constant
      settings: block_version=VER_STRING_GOES_HERE
  SMRO_RxBuff_Radio3 : xbsIndex_r4/Dual Port RAM  depth=2^14  initVector=1:2^14  distributed_mem=Block RAM  init_a=0  init_b=0  rst_a=off  rst_b=off  en_a=off  en_b=off  latency=1  write_mode_A=Read After Write  write_mode_B=Read After Write  dbl_ovrd=off  optimize=Area  use_rpm=on  block_type=dpram
      settings: block_version=VER_STRING_GOES_HERE
  Scope : Scope  NumInputPorts=4
      settings: YMin=-5~-5~-5~-5  YMax=5~5~5~5  SaveName=ScopeData5  MaxDataPoints=50000
  Terminator : Terminator
  Terminator1 : Terminator
  wires:
  SMROWE_RxBuff_Radio3/1 -> SMRO_RxBuff_Radio3/6
  SMRODataI_RxBuff_Radio3/1 -> SMRO_RxBuff_Radio3/5
  Constant/1 -> SMROAddr_RxBuff_Radio3/1
  SMRO_RxBuff_Radio3/2 -> SMRODataO_RxBuff_Radio3/1
  SMROAddr_RxBuff_Radio3/1 -> SMRO_RxBuff_Radio3/4
  SMRO_RxBuff_Radio3/1 -> Terminator/1
  SMRODataO_RxBuff_Radio3/1 -> Terminator1/1
  Addr/1 -> SMRO_RxBuff_Radio3/1, Scope/4
  I/Q/1 -> SMRO_RxBuff_Radio3/2
  Logical/1 -> SMRO_RxBuff_Radio3/3, Scope/1
  WE/1 -> Logical/1, Scope/2
  EN/1 -> Convert1/1, Scope/3
  Convert1/1 -> Logical/2

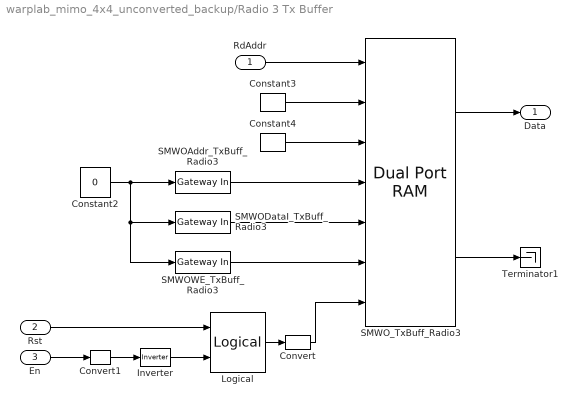
== system warplab_mimo_4x4_unconverted_backup/Radio 3 Tx Buffer ==
  RdAddr : Inport
  Rst : Inport  Port=2
  En : Inport  Port=3
  Constant2 : Constant  Value=0  OutDataType=sfix(16)  ConRadixGroup=Use specified scaling  OutScaling=2^0  SampleTime=inf  FramePeriod=inf
  Constant3 : xbsIndex_r4/Constant  arith_type=Unsigned  const=0  n_bits=32  bin_pt=0  explicit_period=off  period=1  equ=P=C  opselect=C  inp2=PCIN>>17  opr=+  inp1=P  carry=CIN  dbl_ovrd=off  block_type=constant
      settings: block_version=VER_STRING_GOES_HERE
  Constant4 : xbsIndex_r4/Constant  arith_type=Boolean  const=0  n_bits=1  bin_pt=0  explicit_period=off  period=1  equ=P=C  opselect=C  inp2=PCIN>>17  opr=+  inp1=P  carry=CIN  dbl_ovrd=off  block_type=constant
      settings: block_version=VER_STRING_GOES_HERE
  Convert : xbsIndex_r4/Convert  arith_type=Boolean  n_bits=16  bin_pt=14  quantization=Truncate  overflow=Wrap  latency=0  dbl_ovrd=off  pipeline=off  block_type=convert
      settings: block_version=8.2
  Convert1 : xbsIndex_r4/Convert  arith_type=Boolean  n_bits=16  bin_pt=14  quantization=Truncate  overflow=Wrap  latency=0  dbl_ovrd=off  pipeline=off  block_type=convert
      settings: block_version=8.2
  Inverter : xbsIndex_r4/Inverter  en=off  latency=0  dbl_ovrd=off  block_type=inv
      settings: block_version=9.1.01
  Logical : xbsIndex_r4/Logical  logical_function=OR  inputs=2  en=off  latency=0  precision=Full  arith_type=Unsigned  n_bits=16  bin_pt=0  align_bp=on  dbl_ovrd=off  block_type=logical
      settings: block_version=9.1.01
  SMWOAddr_TxBuff_Radio3 : xbsIndex_r4/Gateway In  arith_type=Unsigned  n_bits=14  bin_pt=0  quantization="Round  (unbiased: +/- Inf)"  overflow=Saturate  period=1  dbl_ovrd=off  timing_constraint=None  locs_specified=off  LOCs={}  block_type=gatewayin
      settings: infoedit="Gateway in block.  Converts inputs of type Simulink integer, double and fixed point to  Xilinx fixed point type.<P><P>Hardware notes:  In hardware these blocks become top level input ports."  block_version=VER_STRING_GOES_HERE
  SMWODataI_TxBuff_Radio3 : xbsIndex_r4/Gateway In  arith_type=Unsigned  n_bits=32  bin_pt=0  quantization="Round  (unbiased: +/- Inf)"  overflow=Saturate  period=1  dbl_ovrd=off  timing_constraint=None  locs_specified=off  LOCs={}  block_type=gatewayin
      settings: infoedit="Gateway in block.  Converts inputs of type Simulink integer, double and fixed point to  Xilinx fixed point type.<P><P>Hardware notes:  In hardware these blocks become top level input ports."  block_version=VER_STRING_GOES_HERE
  SMWOWE_TxBuff_Radio3 : xbsIndex_r4/Gateway In  arith_type=Boolean  n_bits=1  bin_pt=0  quantization="Round  (unbiased: +/- Inf)"  overflow=Saturate  period=1  dbl_ovrd=off  timing_constraint=None  locs_specified=off  LOCs={}  block_type=gatewayin
      settings: infoedit="Gateway in block.  Converts inputs of type Simulink integer, double and fixed point to  Xilinx fixed point type.<P><P>Hardware notes:  In hardware these blocks become top level input ports."  block_version=VER_STRING_GOES_HERE
  SMWO_TxBuff_Radio3 : xbsIndex_r4/Dual Port RAM  depth=2^14  initVector=1:2^14  distributed_mem=Block RAM  init_a=0  init_b=0  rst_a=on  rst_b=off  en_a=off  en_b=off  latency=1  write_mode_A=Read After Write  write_mode_B=Read After Write  dbl_ovrd=off  optimize=Area  use_rpm=on  block_type=dpram
      settings: block_version=VER_STRING_GOES_HERE
  Terminator1 : Terminator
  Data : Outport
  wires:
  SMWO_TxBuff_Radio3/1 -> Data/1
  RdAddr/1 -> SMWO_TxBuff_Radio3/1
  Constant2/1 -> SMWOWE_TxBuff_Radio3/1, SMWODataI_TxBuff_Radio3/1, SMWOAddr_TxBuff_Radio3/1
  Constant4/1 -> SMWO_TxBuff_Radio3/3
  Constant3/1 -> SMWO_TxBuff_Radio3/2
  SMWOAddr_TxBuff_Radio3/1 -> SMWO_TxBuff_Radio3/4
  SMWOWE_TxBuff_Radio3/1 -> SMWO_TxBuff_Radio3/6
  SMWODataI_TxBuff_Radio3/1 -> SMWO_TxBuff_Radio3/5
  SMWO_TxBuff_Radio3/2 -> Terminator1/1
  Logical/1 -> Convert/1
  Convert/1 -> SMWO_TxBuff_Radio3/7
  Rst/1 -> Logical/1
  En/1 -> Convert1/1
  Convert1/1 -> Inverter/1
  Inverter/1 -> Logical/2

== system warplab_mimo_4x4_unconverted_backup/Radio 3 Inputs ==
  ADC I : Subsystem
  ADC Q : Subsystem
  Concatenates_1 : Subsystem
  Scope : Scope  NumInputPorts=3
      settings: YMin=-5~-5~-5  YMax=5~5~5
  Radio 3 I/Q : Outport
  wires:
  Concatenates_1/1(32b) -> Radio 3 I/Q/1
  ADC I/1(OTR I) -> Concatenates_1/1(OTR_I)
  ADC I/2(ADC I) -> Scope/1, Concatenates_1/2(ADC_I)
  ADC Q/1(OTR Q) -> Concatenates_1/3(OTR_Q)
  ADC Q/2(ADC Q) -> Scope/2, Concatenates_1/4(ADC_Q)
